simulink model "inverterwithpwm"  (R2017a)
settings: Solver=VariableStepAuto  StartTime=0.0  StopTime=0.1  MaxStep=1e-4  RelTol=1e-3
libraries: powerlib x16, simulink x3, powerlib_meascontrol x3
settings Model: Creator=Bilal Ahmed  LastModifiedBy=Bilal Ahmed

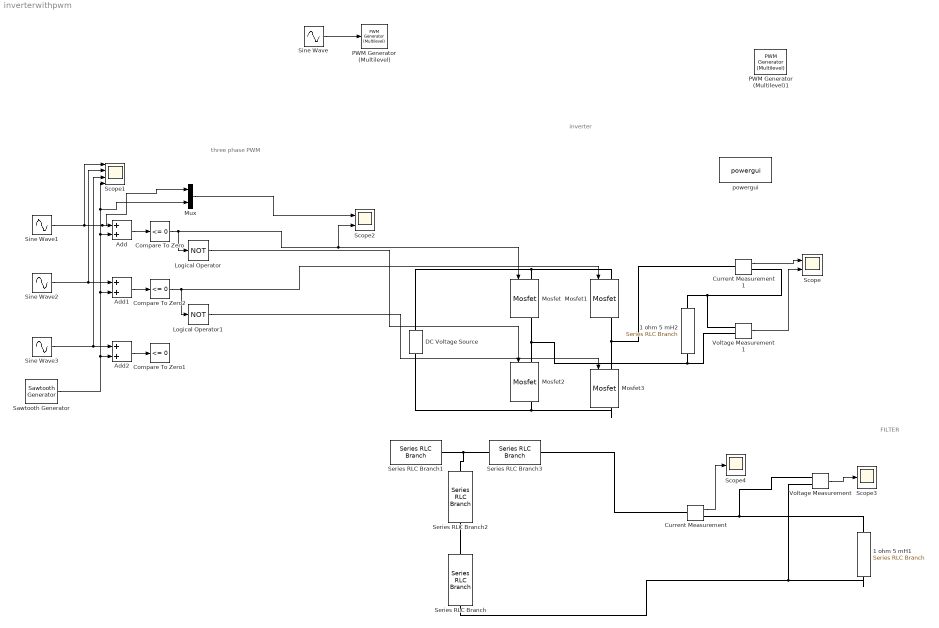
== system inverterwithpwm ==
  note: FILTER
  note: inverter
  note: three phase PWM
  1 ohm 5 mH1 : powerlib/Elements/Series RLC Branch  LConnTagsString=__new0  RConnTagsString=__new0  BranchType=RL  Resistance=1  Inductance=5e-3  SetiL0=off  InitialCurrent=0  Capacitance=400e-6  Setx0=off  InitialVoltage=0  Measurements=None
  1 ohm 5 mH2 : powerlib/Elements/Series RLC Branch  LConnTagsString=__new0  RConnTagsString=__new0  BranchType=R  Resistance=1  Inductance=5e-3  SetiL0=off  InitialCurrent=0  Capacitance=400e-6  Setx0=off  InitialVoltage=0  Measurements=None
  Add : Sum
  Add1 : Sum
  Add2 : Sum
  Compare To Zero : simulink/Logic and Bit Operations/Compare To Zero  relop=<=  OutDataTypeStr=boolean
  Compare To Zero1 : simulink/Logic and Bit Operations/Compare To Zero  relop=<=  OutDataTypeStr=boolean
  Compare To Zero2 : simulink/Logic and Bit Operations/Compare To Zero  relop=<=  OutDataTypeStr=boolean
  Current Measurement : powerlib/Measurements/Current Measurement  PhasorSimulation=off  OutputType=Complex  PSBequivalent=0
  Current Measurement1 : powerlib/Measurements/Current Measurement  PhasorSimulation=off  OutputType=Complex  PSBequivalent=0
  DC Voltage Source : powerlib/Electrical Sources/DC Voltage Source  Amplitude=100  Measurements=Voltage
  Logical Operator : Logic  Operator=NOT  Inputs=1  AllPortsSameDT=off  OutDataTypeStr=boolean
  Logical Operator1 : Logic  Operator=NOT  Inputs=1  AllPortsSameDT=off  OutDataTypeStr=boolean
  Mosfet{,1..3} (4 alike) : powerlib/Power Electronics/Mosfet  Ron=0.1  Lon=0  Rd=0.01  Vfd=0  IC=0  Rs=1e5  Cs=inf  Measurements=on
  Mux : Mux  Inputs=2
  PWM Generator (Multilevel) : powerlib_meascontrol/Pulse & Signal Generators/PWM Generator (Multilevel)  BridgeType=Half-bridge  NumberOfBridges=4  Fc=50  Ts=0  ShowCarriersOutport=off
      settings: SourceProductName=Simscape Power Systems  SourceProductBaseCode=PS
  PWM Generator (Multilevel)1 : powerlib_meascontrol/Pulse & Signal Generators/PWM Generator (Multilevel)  BridgeType=Half-bridge  NumberOfBridges=4  Fc=540  Ts=0  ShowCarriersOutport=off
      settings: SourceProductName=Simscape Power Systems  SourceProductBaseCode=PS
  Sawtooth Generator : powerlib_meascontrol/Pulse & Signal Generators/Sawtooth Generator  Freq=1e3  Phase=180  Ts=0
      settings: SourceProductName=Simscape Power Systems
  Scope : Scope  NumInputPorts=2
  Scope1 : Scope  NumInputPorts=4
  Scope2 : Scope  NumInputPorts=2
  Scope3 : Scope
  Scope4 : Scope
  Series RLC Branch : powerlib/Elements/Series RLC Branch  LConnTagsString=__new0  RConnTagsString=__new0  BranchType=R  Resistance=1.5  Inductance=1e-3  SetiL0=off  InitialCurrent=0  Capacitance=1e-6  Setx0=off  InitialVoltage=0  Measurements=None
  Series RLC Branch1 : powerlib/Elements/Series RLC Branch  LConnTagsString=__new0  RConnTagsString=__new0  BranchType=L  Resistance=1  Inductance=300e-6  SetiL0=off  InitialCurrent=0  Capacitance=1e-6  Setx0=off  InitialVoltage=0  Measurements=None
  Series RLC Branch2 : powerlib/Elements/Series RLC Branch  LConnTagsString=__new0  RConnTagsString=__new0  BranchType=C  Resistance=1  Inductance=1e-3  SetiL0=off  InitialCurrent=0  Capacitance=30e-6  Setx0=off  InitialVoltage=0  Measurements=None
  Series RLC Branch3 : powerlib/Elements/Series RLC Branch  LConnTagsString=__new0  RConnTagsString=__new0  BranchType=L  Resistance=1  Inductance=100e-6  SetiL0=off  InitialCurrent=0  Capacitance=1e-6  Setx0=off  InitialVoltage=0  Measurements=None
  Sine Wave : Sin  Frequency=50  SampleTime=0
  Sine Wave1 : Sin  Frequency=2*pi*50  SampleTime=0
  Sine Wave2 : Sin  Frequency=2*pi*50  Phase=2*pi/3  SampleTime=0
  Sine Wave3 : Sin  Frequency=2*pi*50  Phase=-2*pi/3  SampleTime=0
  Voltage Measurement : powerlib/Measurements/Voltage Measurement  PhasorSimulation=off  OutputType=Complex  PSBequivalent=0
  Voltage Measurement1 : powerlib/Measurements/Voltage Measurement  PhasorSimulation=off  OutputType=Complex  PSBequivalent=0
  powergui : powerlib/powergui  Priority=1  SimulationMode=Continuous  SampleTime=50e-6  frequency=60  Iterations=50  frequencyindice=0  Pbase=100e6  ErrMax=1e-4  UnitsV=kV  UnitsW=MW  buscounter=0  FunctionMessages=off  echomessages=off  EnableUseOfTLC=off  CurrentSourceSwitches=off  DisableSnubberDevices=off  DisableRonSwitches=off  DisableVfSwitches=off  DisplayEquations=off  SolverType=Tustin/Backward Euler (TBE)  Interpol=off  ExternalGateDelay=off  methode=off  Ts=100  x0status=blocks  SPID=on  SwTol=0  HookPort=off  RestoreLinks=warning  ResistiveCurrentMeasurement=off  Frange=[0:2:500]  Ylog=off  Xlog=on  ShowGrid=off  save=off  variable=ZData  structure=0  ZoomFFT=off  StartTime=0.0  cycles=1  DisplayStyle=1  fundamental=60  FreqAxis=off  MaxFrequency=1000  frequencyindicesteady=1  RmsSteady=1  display=off
  wires:
  Sine Wave/1 -> PWM Generator (Multilevel)/1
  Sine Wave1/1 -> Mux/1, Add/1, Scope1/1
  Sine Wave2/1 -> Scope1/2, Add1/1
  Sine Wave3/1 -> Scope1/3, Add2/1
  Sawtooth Generator/1 -> Add2/2, Add1/2, Add/2, Scope1/4, Mux/2
  Add2/1 -> Compare To Zero1/1
  Add1/1 -> Compare To Zero2/1
  Add/1 -> Compare To Zero/1
  Mux/1 -> Scope2/1
  Compare To Zero/1 -> Logical Operator/1, Mosfet/1, Scope2/2
  Compare To Zero2/1 -> Logical Operator1/1, Mosfet1/1
  Voltage Measurement/1 -> Scope3/1
  Logical Operator/1 -> Mosfet2/1
  Logical Operator1/1 -> Mosfet3/1
  Current Measurement/1 -> Scope4/1
  Current Measurement1/1 -> Scope/1
  Voltage Measurement1/1 -> Scope/2
  connections:
  Mosfet/RConn1 -- Voltage Measurement1/LConn2 -- 1 ohm 5 mH2/LConn1 -- Mosfet2/LConn1
  Mosfet/LConn1 -- DC Voltage Source/RConn1 -- Mosfet1/LConn1
  DC Voltage Source/LConn1 -- Mosfet3/RConn1 -- Mosfet2/RConn1
  Series RLC Branch/LConn1 -- 1 ohm 5 mH1/LConn1 -- Voltage Measurement/LConn2
  Series RLC Branch3/LConn1 -- Series RLC Branch2/RConn1 -- Series RLC Branch1/RConn1
  Series RLC Branch3/RConn1 -- Current Measurement/LConn1
  1 ohm 5 mH1/RConn1 -- Voltage Measurement/LConn1 -- Current Measurement/RConn1
  Series RLC Branch/RConn1 -- Series RLC Branch2/LConn1
  Mosfet1/RConn1 -- Current Measurement1/LConn1 -- Mosfet3/LConn1
  1 ohm 5 mH2/RConn1 -- Voltage Measurement1/LConn1 -- Current Measurement1/RConn1
